simulink model "PIDtest"  (R2016a)
settings: Solver=ode45  StartTime=0.0  StopTime=3830  RelTol=1e-3
StartFcn:
  | % clear all
undefined symbols (not defined in the file or in its folder): model_arx, model_bj, model_oe, model_tf
libraries: slident x5, simulink x2, realtime_pacer_lib x1
settings Model: Creator=johnh  LastModifiedBy=tiago
settings DataIOCC: SaveFormat=StructureWithTime
settings OptimizationCC: BlockReduction=off  DefaultParameterBehavior=Inlined  BufferReuse=off
settings HardwareCC: ProdWordSize=32  ProdHWDeviceType=Specified
settings ConfigComp: CovModelRefEnable=Off

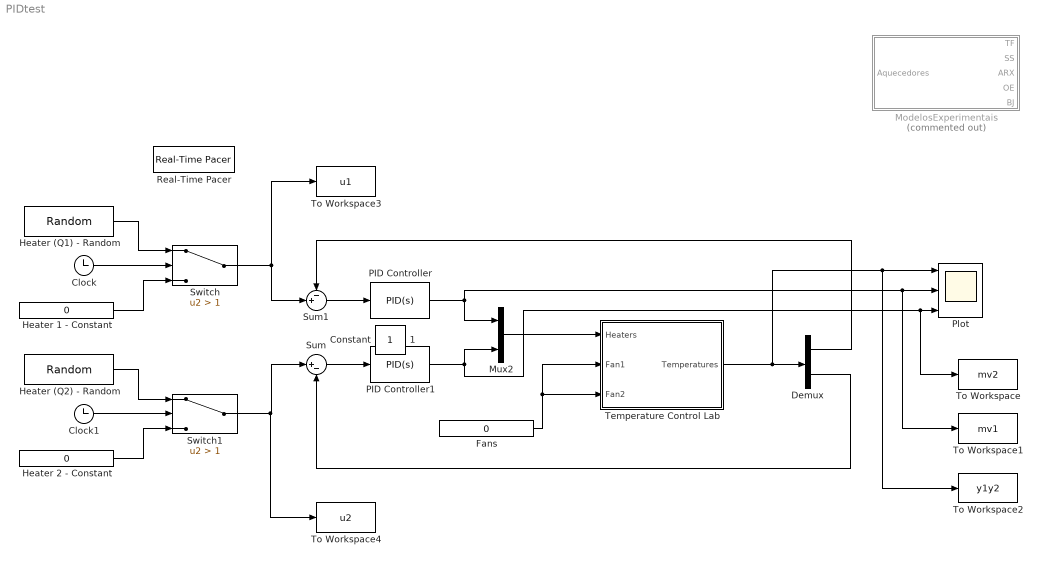
== system PIDtest ==
  Clock : Clock
  Clock1 : Clock
  Demux : Demux  Outputs=2
  Fans : Constant  Value=0
  Heater (Q1) - Random : RandomNumber  Mean=50  Variance=200  Seed=7  SampleTime=766
  Heater (Q2) - Random : RandomNumber  Mean=50  Variance=200  Seed=8  SampleTime=766
  Heater 1 - Constant : Constant  Value=0
  Heater 2 - Constant : Constant  Value=0
  ModelosExperimentais : Subsystem  Commented=on
  Mux2 : Mux  Inputs=2
  PID Controller : simulink/Continuous/PID Controller  Controller=PID  TimeDomain=Continuous-time  SampleTime=-1  IntegratorMethod=Forward Euler  FilterMethod=Forward Euler  Form=Parallel  UseFilter=on  ControllerParametersSource=internal  P=1.43487047389288  I=0.0163886618029911  D=-9.11909332217846  N=0.0216053808675922  InitialConditionSource=internal  InitialConditionForIntegrator=0  InitialConditionForFilter=0  ExternalReset=none  LimitOutput=on  UpperSaturationLimit=100  LowerSaturationLimit=0  LinearizeAsGain=on  AntiWindupMode=none  Kb=1  TrackingMode=off  Kt=1  PParamMin=[]  PParamMax=[]  IParamMin=[]  IParamMax=[]  DParamMin=[]  DParamMax=[]  NParamMin=[]  NParamMax=[]  KbParamMin=[]  KbParamMax=[]  KtParamMin=[]  KtParamMax=[]  POutMin=[]  POutMax=[]  IOutMin=[]  IOutMax=[]  DOutMin=[]  DOutMax=[]  NOutMin=[]  NOutMax=[]  KbOutMin=[]  KbOutMax=[]  KtOutMin=[]  KtOutMax=[]  IntegratorOutMin=[]  IntegratorOutMax=[]  FilterOutMin=[]  FilterOutMax=[]  SumOutMin=[]  SumOutMax=[]  SumI1OutMin=[]  SumI1OutMax=[]  SumI2OutMin=[]  SumI2OutMax=[]  SumI3OutMin=[]  SumI3OutMax=[]  SumDOutMin=[]  SumDOutMax=[]  SaturationOutMin=[]  SaturationOutMax=[]  IntegratorContinuousStateAttributes=''  IntegratorStateMustResolveToSignalObject=off  IntegratorRTWStateStorageClass=Auto  FilterContinuousStateAttributes=''  FilterStateMustResolveToSignalObject=off  FilterRTWStateStorageClass=Auto  DifferentiatorICPrevScaledInput=0  DifferentiatorOutMin=[]  DifferentiatorOutMax=[]
  PID Controller1 : simulink/Continuous/PID Controller  Controller=PID  TimeDomain=Continuous-time  SampleTime=-1  IntegratorMethod=Forward Euler  FilterMethod=Forward Euler  Form=Parallel  UseFilter=on  ControllerParametersSource=internal  P=2.18228807546358  I=0.0111806588363847  D=-30.9190768611892  N=0.00969139842996325  InitialConditionSource=internal  InitialConditionForIntegrator=0  InitialConditionForFilter=0  ExternalReset=none  LimitOutput=on  UpperSaturationLimit=100  LowerSaturationLimit=0  LinearizeAsGain=on  AntiWindupMode=none  Kb=1  TrackingMode=off  Kt=1  PParamMin=[]  PParamMax=[]  IParamMin=[]  IParamMax=[]  DParamMin=[]  DParamMax=[]  NParamMin=[]  NParamMax=[]  KbParamMin=[]  KbParamMax=[]  KtParamMin=[]  KtParamMax=[]  POutMin=[]  POutMax=[]  IOutMin=[]  IOutMax=[]  DOutMin=[]  DOutMax=[]  NOutMin=[]  NOutMax=[]  KbOutMin=[]  KbOutMax=[]  KtOutMin=[]  KtOutMax=[]  IntegratorOutMin=[]  IntegratorOutMax=[]  FilterOutMin=[]  FilterOutMax=[]  SumOutMin=[]  SumOutMax=[]  SumI1OutMin=[]  SumI1OutMax=[]  SumI2OutMin=[]  SumI2OutMax=[]  SumI3OutMin=[]  SumI3OutMax=[]  SumDOutMin=[]  SumDOutMax=[]  SaturationOutMin=[]  SaturationOutMax=[]  IntegratorContinuousStateAttributes=''  IntegratorStateMustResolveToSignalObject=off  IntegratorRTWStateStorageClass=Auto  FilterContinuousStateAttributes=''  FilterStateMustResolveToSignalObject=off  FilterRTWStateStorageClass=Auto  DifferentiatorICPrevScaledInput=0  DifferentiatorOutMin=[]  DifferentiatorOutMax=[]
  Plot : Scope  NumInputPorts=3
  Real-Time Pacer : realtime_pacer_lib/Real-Time Pacer  simTimePerRealTime=1
  Sum : Sum  Inputs=|+-
  Sum1 : Sum  Inputs=-+|
  Switch : Switch  Criteria=u2 > Threshold  Threshold=1
  Switch1 : Switch  Criteria=u2 > Threshold  Threshold=1
  Temperature Control Lab : Subsystem
      mask Display: image('tclab.png');
  To Workspace : ToWorkspace  VariableName=mv2  SaveFormat=Timeseries  SampleTime=-1
  To Workspace1 : ToWorkspace  VariableName=mv1  SaveFormat=Timeseries  SampleTime=-1
  To Workspace2 : ToWorkspace  VariableName=y1y2  SaveFormat=Timeseries  SampleTime=-1
  To Workspace3 : ToWorkspace  VariableName=u1  SaveFormat=Timeseries  SampleTime=-1
  To Workspace4 : ToWorkspace  VariableName=u2  SaveFormat=Timeseries  SampleTime=-1
  1 : Constant  IOType=siggen
  Constant : Constant  IOType=siggen
  wires:
  Sum/1 -> PID Controller1/1
  Sum1/1 -> PID Controller/1
  Demux/2 -> Sum/2
  Demux/1 -> Sum1/1
  Switch1/1 -> To Workspace4/1, Sum/1
  Temperature Control Lab/1(Temperatures) -> To Workspace2/1, Plot/1, Demux/1
  Mux2/1 -> Temperature Control Lab/1(Heaters)
  Fans/1 -> Temperature Control Lab/2(Fan1), Temperature Control Lab/3(Fan2)
  PID Controller/1 -> Mux2/1, To Workspace1/1, Plot/2
  PID Controller1/1 -> Mux2/2, To Workspace/1, Plot/3
  Heater (Q1) - Random/1 -> Switch/1
  Clock/1 -> Switch/2
  Heater 1 - Constant/1 -> Switch/3
  Heater (Q2) - Random/1 -> Switch1/1
  Clock1/1 -> Switch1/2
  Heater 2 - Constant/1 -> Switch1/3
  Switch/1 -> Sum1/2, To Workspace3/1

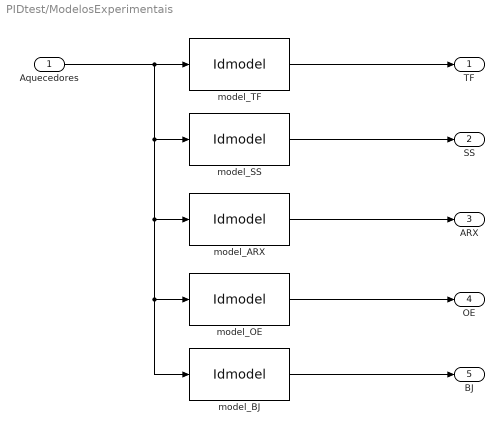
== system PIDtest/ModelosExperimentais ==
  Aquecedores : Inport
  model_ARX : slident/Models/Idmodel  sys=model_arx.model{1,1}  IC=0  noi=on  seed=[]
  model_BJ : slident/Models/Idmodel  sys=model_bj.model{1,1}  IC=0  noi=on  seed=[]
  model_OE : slident/Models/Idmodel  sys=model_oe.model{1,1}  IC=0  noi=on  seed=[]
  model_SS : slident/Models/Idmodel  sys=model_ss  IC=0  noi=on  seed=[]
  model_TF : slident/Models/Idmodel  sys=model_tf.model{1,1}  IC=0  noi=on  seed=[]
  TF : Outport
  SS : Outport  Port=2
  ARX : Outport  Port=3
  OE : Outport  Port=4
  BJ : Outport  Port=5
  wires:
  Aquecedores/1 -> model_BJ/1, model_OE/1, model_ARX/1, model_SS/1, model_TF/1
  model_TF/1 -> TF/1
  model_SS/1 -> SS/1
  model_ARX/1 -> ARX/1
  model_OE/1 -> OE/1
  model_BJ/1 -> BJ/1

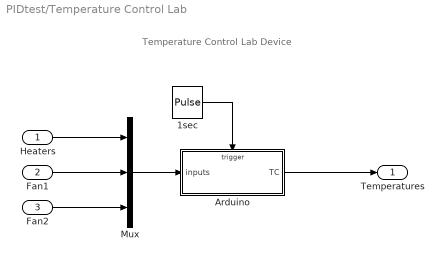
== system PIDtest/Temperature Control Lab ==
  note: Temperature Control Lab Device
  Heaters : Inport  PortDimensions=2
  Fan1 : Inport  Port=2  PortDimensions=1
  Fan2 : Inport  Port=3  PortDimensions=1
  1sec : DiscretePulseGenerator  PulseType=Time based  Period=0.5  PulseWidth=50
  Arduino : Subsystem  TreatAsAtomicUnit=on
  Mux : Mux  Inputs=3
  Temperatures : Outport
  wires:
  1sec/1 -> Arduino/Trigger
  Arduino/1(TC) -> Temperatures/1
  Mux/1 -> Arduino/1(inputs)
  Heaters/1 -> Mux/1
  Fan2/1 -> Mux/3
  Fan1/1 -> Mux/2

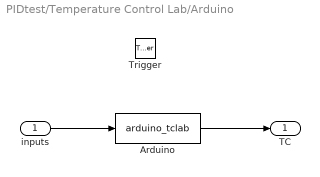
== system PIDtest/Temperature Control Lab/Arduino ==
  inputs : Inport  PortDimensions=4  LatchByDelayingOutsideSignal=on
  Trigger : TriggerPort  VariantControl=Variant
  Arduino : MATLABFcn  MATLABFcn=arduino_tclab
  TC : Outport  InitialOutput=[23 23]
  wires:
  inputs/1 -> Arduino/1
  Arduino/1 -> TC/1
